simulink model "LAB2_"  (R2025b)
settings: Solver=FixedStepDiscrete  StartTime=0.0  StopTime=10  FixedStep=T  RelTol=1e-3
undefined symbols (not defined in the file): daq, den_Hi, DiscIntNeverNeededParam, Kd, Kp, mot, National_Instruments, num_Hi, PCI, sens, T, Tl
libraries: sldrtlib x3
settings Model: SimulationMode=external  ExtModeTrigDuration=100001  Creator=delpratogi  LastModifiedBy=Gioele
settings DataIOCC: ReturnWorkspaceOutputs=off
settings HardwareCC: ProdBitPerLong=64.0  ProdHWDeviceType=Intel->x86-64 (Linux 64)
settings RTWCC: SystemTargetFile=sldrt.tlc  TemplateMakefile=sldrt.tmf  RTWCompilerOptimization=on  Description=Simulink Desktop Real-Time
settings CodeAppCC: MaxIdLength=95.0
settings SimulinkDesktopRealTimeCC: ExtModeTransport=0.0  ExtModeStaticAllocSize=1000000.0  TargetLibSuffix=_sldrt.a  TargetPreCompLibLocation=C:\Program Files\MATLAB\R2025b\toolbox\sldrt\lib\win64  MultiwordLength=2048.0  DynamicStringBufferSize=256.0  ParMdlRefBuildCompliant=on  PreserveMATLABNamespacesInGeneratedCode=on  SubcomponentCodeInterfacePackaging=Reusable function  SupportVariableSizeSignals=off

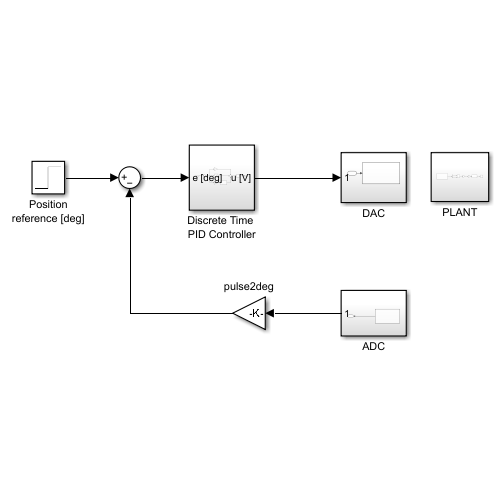
[thumbnail: Simulink's stored preview of the top-level diagram]
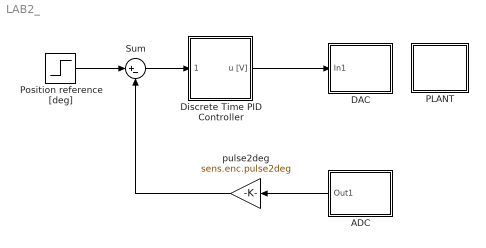
== system LAB2_ ==
  ADC : Subsystem
  DAC : Subsystem
  Discrete Time PID Controller : Subsystem
  PLANT : Subsystem
  Position reference [deg] : Step  Time=0  After=50  SampleTime=T
  Sum : Sum  Inputs=|+-
  pulse2deg : Gain  Gain=sens.enc.pulse2deg
  wires:
  Position reference [deg]/1 -> Sum/1
  Sum/1 -> Discrete Time PID Controller/1(e [deg])
  pulse2deg/1 -> Sum/2
  Discrete Time PID Controller/1(u [V]) -> DAC/1(In1)
  ADC/1(Out1) -> pulse2deg/1

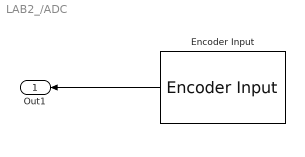
== system LAB2_/ADC ==
  Encoder Input : sldrtlib/Encoder Input  SampleTime=0.001  MaxMissedTicks=10  ShowMissedTicks=off  YieldWhenWaiting=off  DrvName=National_Instruments/PCI-6221  DrvAddress=4294967295  DrvOptions=[0 0 0 2 0]  Channels=1  QuadMode=3  IndexPulse=1  InputFilter=Inf  DataType=1
      settings: AttributesFormatString=National Instruments\nPCI-6221 [auto]
  Out1 : Outport
  wires:
  Encoder Input/1 -> Out1/1

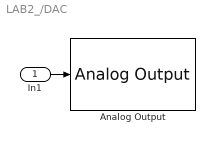
== system LAB2_/DAC ==
  In1 : Inport
  Analog Output : sldrtlib/Analog Output  SampleTime=0.001  MaxMissedTicks=10  ShowMissedTicks=off  YieldWhenWaiting=off  DrvName=National_Instruments/PCI-6221  DrvAddress=4294967295  DrvOptions=[0 0 0 2 0]  Channels=1  RangeMode=1  VoltRange=1  InitialValue=0  FinalValue=0
      settings: AttributesFormatString=National Instruments\nPCI-6221 [auto]
  wires:
  In1/1 -> Analog Output/1

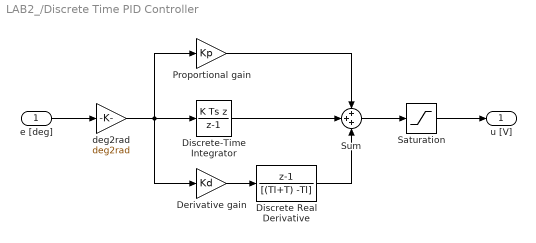
== system LAB2_/Discrete Time PID Controller ==
  e [deg] : Inport
  Derivative gain : Gain  Gain=Kd
  Discrete Real Derivative : DiscreteTransferFcn  Numerator=[1 -1]  Denominator=[(Tl+T) -Tl]
  Discrete-Time Integrator : DiscreteIntegrator  IntegratorMethod=Integration: Backward Euler  gainval=Ki  SampleTime=T  ICPrevOutput=DiscIntNeverNeededParam  ICPrevScaledInput=DiscIntNeverNeededParam
  Proportional gain : Gain  Gain=Kp
  Saturation : Saturate  UpperLimit=daq.dac.fs  LowerLimit=-daq.dac.fs
  Sum : Sum  Inputs=+++
  deg2rad : Gain  Gain=deg2rad
  u [V] : Outport
  wires:
  Discrete Real Derivative/1 -> Sum/3
  Proportional gain/1 -> Sum/1
  e [deg]/1 -> deg2rad/1
  Sum/1 -> Saturation/1
  Saturation/1 -> u [V]/1
  deg2rad/1 -> Discrete-Time Integrator/1, Proportional gain/1, Derivative gain/1
  Derivative gain/1 -> Discrete Real Derivative/1
  Discrete-Time Integrator/1 -> Sum/2

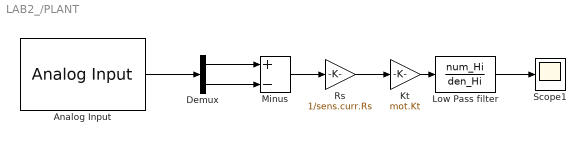
== system LAB2_/PLANT ==
  Analog Input : sldrtlib/Analog Input  SampleTime=0.001  MaxMissedTicks=10  ShowMissedTicks=off  YieldWhenWaiting=off  DrvName=National_Instruments/PCI-6221  DrvAddress=4294967295  DrvOptions=[0 0 0 2 0]  Channels=[1,2]  RangeMode=1  VoltRange=1  DataType=1
      settings: AttributesFormatString=National Instruments\nPCI-6221 [auto]
  Demux : Demux  Outputs=2
  Kt : Gain  Gain=mot.Kt
  Low Pass filter : TransferFcn  Numerator=num_Hi  Denominator=den_Hi
  Minus : Sum  Inputs=+-
  Rs : Gain  Gain=1/sens.curr.Rs
  Scope1 : Scope
  wires:
  Low Pass filter/1 -> Scope1/1
  Demux/1 -> Minus/1
  Minus/1 -> Rs/1
  Analog Input/1 -> Demux/1
  Kt/1 -> Low Pass filter/1
  Demux/2 -> Minus/2
  Rs/1 -> Kt/1
